simulink model "DA1"  (Simulink 8.7)
settings: Solver=ode45  StartTime=0.0  StopTime=300  RelTol=1e-3
settings Model: Creator=mwwhalen  LastModifiedBy=bourbouh
settings DataIOCC: ExternalInput=[t,u]  SignalLoggingSaveFormat=ModelDataLogs
settings OptimizationCC: ExpressionDepthLimit=2147483647  InitFltsAndDblsToZero=on
settings DebuggingCC: SaveWithParameterizedLinksMsg=none  SignalResolutionControl=TryResolveAllWithWarning  SolverPrmCheckMsg=warning  MultiTaskDSMMsg=warning  MultiTaskCondExecSysMsg=none  FcnCallInpInsideContextMsg=UseLocalSettings  StateNameClashWarn=warning  StrictBusMsg=None
settings SFSimCC: SimParseCustomCode=off
settings GRTTargetCC: TargetFcnLib=ansi_tfl_tmw.mat  CombineOutputUpdateFcns=off  GRTInterface=on

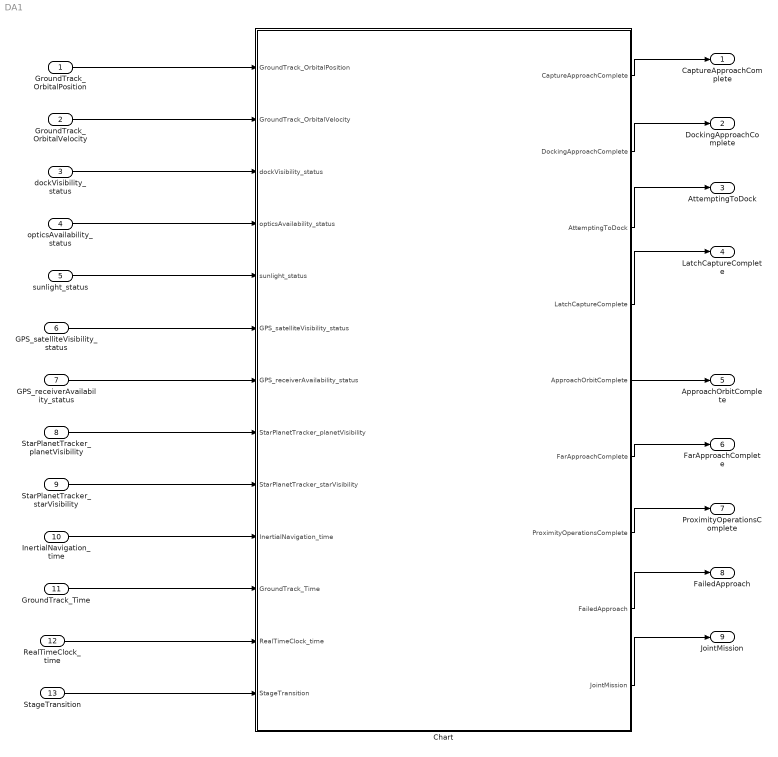
== system DA1 ==
  GroundTrack_OrbitalPosition : Inport
  GroundTrack_OrbitalVelocity : Inport  Port=2
  dockVisibility_status : Inport  Port=3
  opticsAvailability_status : Inport  Port=4
  sunlight_status : Inport  Port=5
  GPS_satelliteVisibility_status : Inport  Port=6
  GPS_receiverAvailability_status : Inport  Port=7
  StarPlanetTracker_planetVisibility : Inport  Port=8
  StarPlanetTracker_starVisibility : Inport  Port=9
  InertialNavigation_time : Inport  Port=10
  GroundTrack_Time : Inport  Port=11
  RealTimeClock_time : Inport  Port=12
  StageTransition : Inport  Port=13
  Chart : Stateflow chart  TreatAsAtomicUnit=on
  CaptureApproachComplete : Outport
  DockingApproachComplete : Outport  Port=2
  AttemptingToDock : Outport  Port=3
  LatchCaptureComplete : Outport  Port=4
  ApproachOrbitComplete : Outport  Port=5
  FarApproachComplete : Outport  Port=6
  ProximityOperationsComplete : Outport  Port=7
  FailedApproach : Outport  Port=8
  JointMission : Outport  Port=9
  wires:
  GroundTrack_OrbitalVelocity/1 -> Chart/2(GroundTrack_OrbitalVelocity)
  dockVisibility_status/1 -> Chart/3(dockVisibility_status)
  opticsAvailability_status/1 -> Chart/4(opticsAvailability_status)
  sunlight_status/1 -> Chart/5(sunlight_status)
  GPS_satelliteVisibility_status/1 -> Chart/6(GPS_satelliteVisibility_status)
  StarPlanetTracker_planetVisibility/1 -> Chart/8(StarPlanetTracker_planetVisibility)
  StarPlanetTracker_starVisibility/1 -> Chart/9(StarPlanetTracker_starVisibility)
  InertialNavigation_time/1 -> Chart/10(InertialNavigation_time)
  GroundTrack_Time/1 -> Chart/11(GroundTrack_Time)
  RealTimeClock_time/1 -> Chart/12(RealTimeClock_time)
  GroundTrack_OrbitalPosition/1 -> Chart/1(GroundTrack_OrbitalPosition)
  StageTransition/1 -> Chart/13(StageTransition)
  GPS_receiverAvailability_status/1 -> Chart/7(GPS_receiverAvailability_status)
  Chart/2(DockingApproachComplete) -> DockingApproachComplete/1
  Chart/1(CaptureApproachComplete) -> CaptureApproachComplete/1
  Chart/3(AttemptingToDock) -> AttemptingToDock/1
  Chart/4(LatchCaptureComplete) -> LatchCaptureComplete/1
  Chart/5(ApproachOrbitComplete) -> ApproachOrbitComplete/1
  Chart/6(FarApproachComplete) -> FarApproachComplete/1
  Chart/7(ProximityOperationsComplete) -> ProximityOperationsComplete/1
  Chart/8(FailedApproach) -> FailedApproach/1
  Chart/9(JointMission) -> JointMission/1

== stateflow chart Chart ==
  settings: updateMethod=DISCRETE  sampleTime=1
  state MissionPhaseStates [parallel]
    settings: executionOrder=1
    state FarApproach
    state JointStabilize
    state Start /
    state DockingApproach
    state CollisionAvoidanceManuever/
      exit:
      ApproachOrbitComplete=0;
      ProximityOperationsComplete=0;
      FarApproachComplete=0;
      CaptureApproachComplete= 0;
    state ApproachOrbit
    state Disengage
    state ProximityOperations
    state JointMission /
      entry: JointMission=1;
    state CaptureApproach
    state LatchCapture
      state LatchCaptureCheck / [parallel]
        entry:AttemptingToDock = 1;
        during:LatchCapture_timer = min(LatchCapture_timer + 1,LatchCapture_timer_upper_limit+1/*9*/);
        exit : AttemptingToDock = 0;
        settings: executionOrder=1
        state Docked
          entry:LatchCaptureComplete = 1;
        state LatchFailed
        state CheckLatchOpen /
          entry : LatchCapture_timer = 0;
        state CheckLatchMated
        (default) -> CheckLatchOpen 
        CheckLatchOpen  -> CheckLatchMated [order 1] : [latch_status == OPEN]
        CheckLatchMated -> Docked [order 1] : [latch_status == MATED]
        CheckLatchMated -> (junction 49) [order 3] : [LatchCapture_timer == LatchCapture_timer_upper_limit/*9*/]
        CheckLatchMated -> (junction 49) [order 2] : [latch_status == CLOSEDBUTUNMATED]
        CheckLatchOpen  -> LatchFailed [order 2] : [LatchCapture_timer == LatchCapture_timer_upper_limit/*9*/]
        (junction 49) -> LatchFailed
      state latch [parallel]
        settings: executionOrder=2
        state ClosedButUnmated /
          entry : latch_status = CLOSEDBUTUNMATED
        state Open /
          entry : latch_status = OPEN
        state Closing /
          entry : latch_status = INDETERMINATE
        state Mated /
          entry : latch_status = MATED
        state Opening /
          entry : latch_status = INDETERMINATE
        (default) -> Opening 
        (junction 57) -> Opening 
        Opening  -> Closing  [order 2] : /*closeLatch*/
        Opening  -> Open  [order 1] : /*open*/
        Open  -> Closing  : /*closeLatch*/
        Closing  -> ClosedButUnmated  [order 3] : /*closedButUnmated*/
        Closing  -> Mated  [order 1] : /*mated*/
        Closing  -> (junction 57) [order 2] : /*openLatch*/
        Mated  -> (junction 57) : /*openLatch*/
        ClosedButUnmated  -> (junction 57)
    state FailedApproach /
      entry: FailedApproach=1;
    (default) -> Start 
    Start  -> ApproachOrbit : [StageTransition == 0
        | /*Approach*/]
    CollisionAvoidanceManuever -> ApproachOrbit [order 2] : [StageTransition == 6]
        | /*isSafeToApproach*/
    ProximityOperations -> ApproachOrbit [order 1] : [StageTransition == 1]
        | {ApproachOrbitComplete=0;}
        | /*FailedProximityApproach*/
    ApproachOrbit -> ProximityOperations : [StageTransition == 2]
        | {ApproachOrbitComplete=1}
        |  /*isInSameOrbit*/
    FarApproach -> CollisionAvoidanceManuever [order 1] : [StageTransition == 5]
        | /*FailedFarApproach*/
    CaptureApproach -> CollisionAvoidanceManuever [order 2]
    Disengage -> CollisionAvoidanceManuever : [StageTransition == 7]
        | /*isDisengaged*/
    CollisionAvoidanceManuever -> FailedApproach  [order 1] : [StageTransition == 8]
        | /*FailedApproach*/
    ProximityOperations -> FarApproach [order 2] : [StageTransition == 3]
        | {ProximityOperationsComplete=1}
        | /*isInSight*/
    JointStabilize -> Disengage [order 1] : [ StageTransition == 9]
        | /*LatchLost*/
    FarApproach -> CaptureApproach [order 2] : [StageTransition == 4]
        | {FarApproachComplete=1}
        | /*InProximity*/
    JointStabilize -> JointMission  [order 2] : [StageTransition == 10]
        | /*JointMission*/
    DockingApproach -> CaptureApproach [order 2] : /*DockingApproachFailed*/
    CaptureApproach -> DockingApproach [order 1] : [StageTransition==5]
        | {CaptureApproachComplete = 1}
    DockingApproach -> LatchCapture [order 1] : [StageTransition == 6]
        | {DockingApproachComplete = 1}
    Docked -> JointStabilize : /*Docked*/
    LatchFailed -> DockingApproach : /*LatchFailed*/
  data: INDETERMINATE constant int8; OPEN constant int8 =1; CLOSEDBUTUNMATED constant int8 =2; MATED constant int8 =3; EXIST constant boolean =1; AVAILABLE constant boolean =1; EXPIRED constant boolean =1; NONE constant int8; POOR constant int8 =1; GOOD constant int8 =2; GroundTrack_OrbitalPosition input int8; GroundTrack_OrbitalVelocity input int8; dockVisibility_status input int8; opticsAvailability_status input boolean; sunlight_status input boolean; GPS_satelliteVisibility_status input int8; GPS_receiverAvailability_status input boolean; StarPlanetTracker_planetVisibility input int8; StarPlanetTracker_starVisibility input int8; InertialNavigation_time input boolean; GroundTrack_Time input int8; latch_status local int8; LatchCapture_timer local int8; RealTimeClock_time input int8; BRIGHT constant boolean =1; StageTransition input int8; CaptureApproach_timer_upper_limit constant int8 =11; CaptureApproachComplete output boolean; DockingApproachComplete output boolean; AttemptingToDock output boolean; LatchCaptureComplete output boolean; ApproachOrbitComplete output boolean; FarApproachComplete output boolean; ProximityOperationsComplete output boolean; FailedApproach output boolean; JointMission output boolean; StarPlanetTracker_timer_upper_limit constant int8 =6; InertialNavigation_timer_upper_limit constant int8 =6; GPS_timer_upper_limit constant int8 =6; DockingApproach_timer_upper_limit constant int8 =9; dockingSensor_timer_upper_limit constant int8 =6; LatchCapture_timer_upper_limit constant int8 =8
